simulink model "Fuel_Cell_IV_Curve"  (R2021a)
settings: Solver=VariableStepAuto  StartTime=0.0  StopTime=Tsim  RelTol=1e-3
InitFcn:
  | V_init = 10;
values from neighbouring files (symbols this model uses):
  FinalVoltage = 25    [demo_script_IV.m]
  InitVoltage = 50    [demo_script_IV.m]
  xI = x_vect(i)    [demo_script_IV.m]
  xOC = 1    [demo_script_IV.m]
  xR = 1    [demo_script_IV.m]
undefined symbols (not defined in the file or in its folder): FuelCell
libraries: fl_lib x12, nesl_utility x4, ee_lib x2
settings Model: Creator=jsagardu  LastModifiedBy=LENOVO
settings SolverCC: AlgebraicLoopSolver=TrustRegion
settings DataIOCC: ReturnWorkspaceOutputs=off
settings DebuggingCC: SymbolicDimsDataTypeCodeGenerationDiagnostic=none  SFMachineParentedDataDiag=warning
settings SFSimCC: CustomCodeUndefinedFunction=UseInterfaceOnly
settings SimscapeCC: SimscapeLogType=local  SimscapeLogLimitData=off  SimscapeLogDataHistory=10000

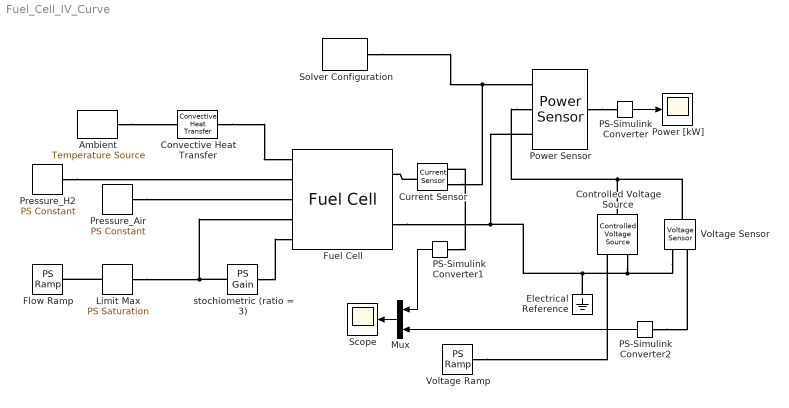
== system Fuel_Cell_IV_Curve ==
  Ambient : fl_lib/Thermal/Thermal Sources/Temperature Source  temperature=293.15 K
  Controlled Voltage Source : fl_lib/Electrical/Electrical Sources/Controlled Voltage Source
  Convective Heat Transfer : fl_lib/Thermal/Thermal Elements/Convective Heat Transfer  area=120 cm^2  heat_tr_coeff=20 W/(m^2 * K)  T_specify=off  T_priority=None  T=0 K  T_nominal_specify=off  T_nominal_unit=K  T_nominal_value=1  Q_specify=off  Q_priority=None  Q=0 W  Q_nominal_specify=off  Q_nominal_unit=W  Q_nominal_value=1
  Current Sensor : fl_lib/Electrical/Electrical Sensors/Current Sensor
  Electrical Reference : fl_lib/Electrical/Electrical Elements/Electrical Reference
  Flow Ramp : fl_lib/Physical Signals/Sources/PS Ramp  slope=100/360 lpm/s  start_time=Tstart s  initial_output=FuelCell.Init_Qfuel lpm
      settings: SourceProductBaseCode=SS
  Fuel Cell : ee_lib/Sources/Fuel Cell  model_fidelity=ee.enum.fuelcell.fidelity.detailed  Eoc=FuelCell.OpenCircuitVoltage*xOC V  A=FuelCell.TafelSlope V  ri=FuelCell.InternalResistance*xR Ohm  i0=FuelCell.NomExchangeCurrent*xI A  N_cell=65  number_unit=Nu  dyn=ee.enum.include.no  i_lim=FuelCell.CollapseCurrent*xI A  Tnom=293.15 K  thermal_mass=15000 J/K  pH2_nom=FuelCell.NomH2_Pressure Pa  pO2_nom=FuelCell.NomAir_Pressure Pa  xH2=99  xO2=21  xW=0  Rd=0.005 Ohm  tau=10 s  iFC_specify=off  iFC_priority=High  iFC=10 A  iFC_nominal_specify=off  iFC_nominal_unit=A  iFC_nominal_value=1  vFC_specify=on  vFC_priority=High  vFC=FuelCell.InitVoltage V  vFC_nominal_specify=off  vFC_nominal_unit=V  vFC_nominal_value=1  temperature_specify=off  temperature_priority=High  temperature=293 K  temperature_nominal_specify=off  temperature_nominal_unit=K  temperature_nominal_value=1
      settings: SourceProductBaseCode=PS  LogSimulationData=on  InternalSimscapePortConfiguration="{\"Bottom\":[],\"Left\":[{\"id\":\"H\",\"label\":\"H\",\"type\":\"foundation.thermal.thermal\"},{\"id\":\"pfuel\",\"label\":\"pfuel\",\"type\":\"input\"},{\"id\":\"pair\",\"label\":\"pair\",\"type\":\"input\"},{\"id\":\"qfuel\",\"label\":\"qfuel\",\"type\":\"input\"},{\"id\":\"qair\",\"label\":\"qair\",\"type\":\"input\"}],\"Right\":[{\"id\":\"p\",\"label\":\"+\",\"type\":\"foundation.electrical.electrical\"},{\"id\":\"n\",\"label\":\"-\",\"type\":\"foundation.electrical.electrical\"}],\"Top\":[]}"
  Limit Max : fl_lib/Physical Signals/Nonlinear Operators/PS Saturation  upper_limit=100 lpm  lower_limit=0 lpm
      settings: SourceProductBaseCode=SS
  Mux : Mux  Inputs=2
  PS-Simulink Converter : nesl_utility/PS-Simulink Converter  PhysicalDomain=network_engine_domain  SubClassName=ps_output  LeftPortType=input  RightPortType=output  PseudoPeriodic=off  Frequencies=[]  Unit=kW  AffineConversion=off
      settings: SourceProductName=Utilities
  PS-Simulink Converter1 : nesl_utility/PS-Simulink Converter  PhysicalDomain=network_engine_domain  SubClassName=ps_output  LeftPortType=input  RightPortType=output  PseudoPeriodic=off  Frequencies=[]  Unit=inherit  AffineConversion=off
      settings: SourceProductBaseCode=PW,SS
  PS-Simulink Converter2 : nesl_utility/PS-Simulink Converter  PhysicalDomain=network_engine_domain  SubClassName=ps_output  LeftPortType=input  RightPortType=output  PseudoPeriodic=off  Frequencies=[]  Unit=inherit  AffineConversion=off
      settings: SourceProductBaseCode=PW,SS
  Power Sensor : ee_lib/Sensors & Transducers/Power Sensor  measurement_type=1  averaging_period=1e-4 s
      settings: SourceProductBaseCode=PS  LogSimulationData=on
  Power [kW] : Scope
  Pressure_Air : fl_lib/Physical Signals/Sources/PS Constant  constant=1.0 bar
  Pressure_H2 : fl_lib/Physical Signals/Sources/PS Constant  constant=pH2 bar
      settings: AttributesFormatString=[2.5 - 5.0] bar
  Scope : Scope
  Solver Configuration : nesl_utility/Solver Configuration  PhysicalDomain=network_engine_domain  SubClassName=solver  LeftPortType=input  RightPortType=generic  Tones=[]  Harmonics=[]  SimulateNoise=off  Profile=off  UseLocalSampling=off  EnableSwitchedLinearOptims=on  FrequencyDomain=off  UseCCode=off  RelTol=0.001  AbsTol=1e-06  MinStep=1e-09  ToWorkspace=off  RevertToSquareIcSolve=off  NumHomotopyIterations=100  PhasorMode=off  PhasorModeNumHarmonics=1  DoDC=off  ResidualTolerance=1e-09  UseLocalSolver=off  LocalSolverChoice=NE_BACKWARD_EULER_ADVANCER  LocalSolverSampleTime=0.001  DoFixedCost=off  MaxNonlinIter=3  MaxModeIter=2  ComputeImpulses=off  ImpulseIterations=2  LinearAlgebra=auto  EquationFormulation=NE_TIME_EF  DelaysMemoryBudget=1024  AutomaticFiltering=on  FilteringTimeConstant=0.001  PartitionStorageMethod=AS_NEEDED  PartitionMemoryBudget=1024  PartitionMethod=ROBUST
      settings: SourceProductName=Utilities
  Voltage Ramp : fl_lib/Physical Signals/Sources/PS Ramp  slope=(FinalVoltage-InitVoltage)/360 V/s  start_time=Tstart s  initial_output=InitVoltage V
      settings: SourceProductBaseCode=SS
  Voltage Sensor : fl_lib/Electrical/Electrical Sensors/Voltage Sensor
  stochiometric (ratio = 3) : fl_lib/Physical Signals/Functions/PS Gain  gain=3.0
  wires:
  PS-Simulink Converter/1 -> Power [kW]/1
  Mux/1 -> Scope/1
  PS-Simulink Converter1/1 -> Mux/1
  PS-Simulink Converter2/1 -> Mux/2
  connections:
  Controlled Voltage Source/RConn2 -- Voltage Sensor/RConn2 -- Electrical Reference/LConn1 -- Fuel Cell/RConn2 -- Power Sensor/LConn3
  Solver Configuration/RConn1 -- Current Sensor/RConn2 -- Power Sensor/LConn1
  Power Sensor/LConn2 -- Controlled Voltage Source/LConn1 -- Voltage Sensor/LConn1
  Power Sensor/RConn1 -- PS-Simulink Converter/LConn1
  Pressure_Air/RConn1 -- Fuel Cell/LConn3
  Convective Heat Transfer/LConn1 -- Fuel Cell/LConn1
  Ambient/LConn1 -- Convective Heat Transfer/RConn1
  Limit Max/RConn1 -- stochiometric (ratio = 3)/LConn1 -- Fuel Cell/LConn4
  Limit Max/LConn1 -- Flow Ramp/RConn1
  stochiometric (ratio = 3)/RConn1 -- Fuel Cell/LConn5
  Current Sensor/LConn1 -- Fuel Cell/RConn1
  PS-Simulink Converter1/LConn1 -- Current Sensor/RConn1
  PS-Simulink Converter2/LConn1 -- Voltage Sensor/RConn1
  Pressure_H2/RConn1 -- Fuel Cell/LConn2
  Voltage Ramp/RConn1 -- Controlled Voltage Source/RConn1
